simulink model "untitled1"  (R2024b)
settings: Solver=VariableStepAuto  StartTime=0.0  StopTime=10.0  RelTol=1e-3
model workspace (MAT data in the model file):
  Lm = 0
  Lr = 0
  Ls = 0
undefined symbols (not defined in the file): lr
settings Model: Creator=antoinedaniel  LastModifiedBy=antoinedaniel

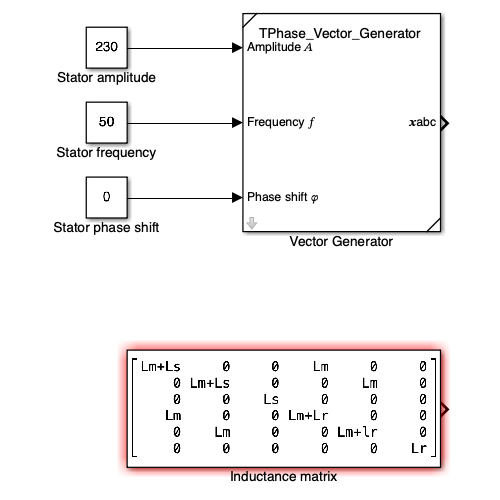
[thumbnail: Simulink's stored preview of the top-level diagram]
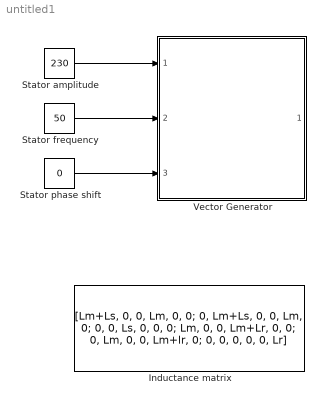
== system untitled1 ==
  Inductance matrix : Constant  Value=[Lm+Ls, 0, 0, Lm, 0, 0; 0, Lm+Ls, 0, 0, Lm, 0; 0, 0, Ls, 0, 0, 0; Lm, 0, 0, Lm+Lr, 0, 0; 0, Lm, 0, 0, Lm+lr, 0; 0, 0, 0, 0, 0, Lr]
  Stator amplitude : Constant  Value=230
  Stator frequency : Constant  Value=50
  Stator phase shift : Constant  Value=0
  Vector Generator : Subsystem  ReferencedSubsystem=TPhase_Vector_Generator
  wires:
  Stator amplitude/1 -> Vector Generator/1
  Stator frequency/1 -> Vector Generator/2
  Stator phase shift/1 -> Vector Generator/3
